simulink model "player_ball_5"  (R2021b)
settings: Solver=VariableStepAuto  StartTime=0.0  StopTime=300  RelTol=1e-3
model workspace (MAT data in the model file):
  trailfuzzy = 'trailfuzzy.fis'
values from neighbouring files (symbols this model uses):
  initBallPos = fieldCenter    [robotSoccerParams.m]
  robotDetectorMaxHits = 5    [robotSoccerParams.m]
  sampleTime = 0.05    [robotSoccerParams.m]
undefined symbols (not defined in the file or in its folder): DiscIntNeverNeededParam
libraries: mobileRoboticsLib x11, dspindex x3, fuzblock x2
settings Model: Creator=kstkr  LastModifiedBy=kstkr
settings DebuggingCC: AlgebraicLoopMsg=none

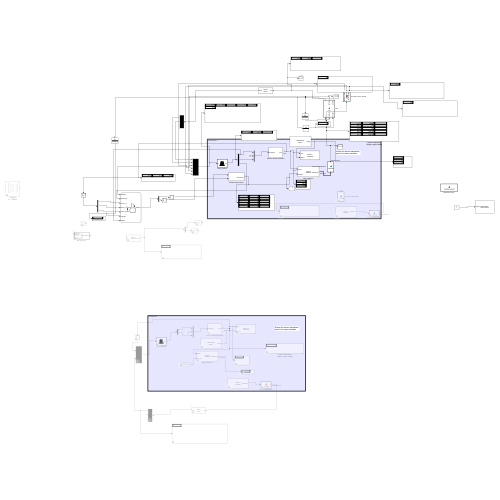
[thumbnail: Simulink's stored preview of the top-level diagram]
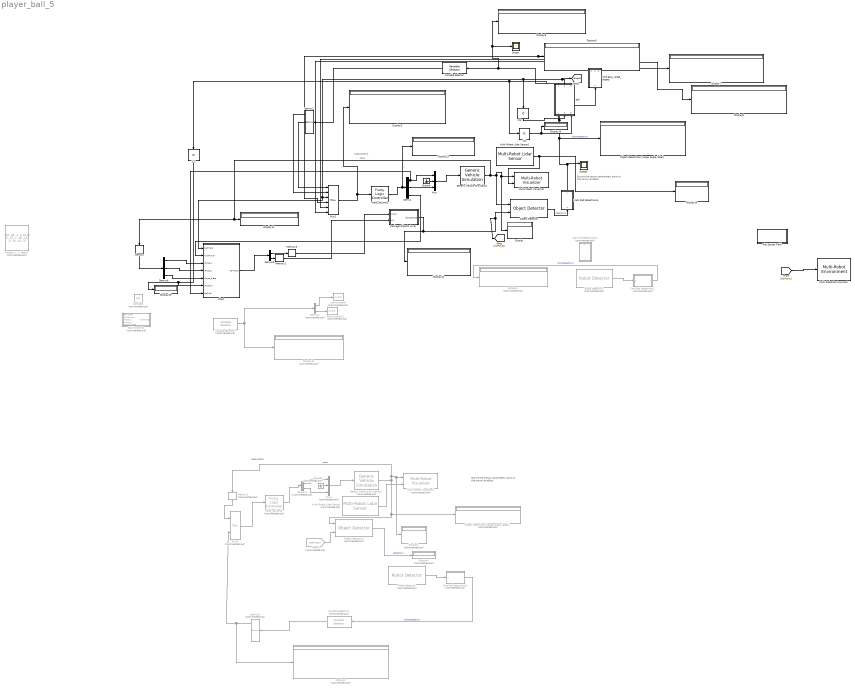
== system player_ball_5 ==
  note: Subsystem1
  note: Subsystem
  note: Ensure the sensor parameters point to the same variables.
  note: Ensure the sensor parameters point to the same variables.
  Add Constant : Bias  Commented=on  Bias=0.3
  Add Constant1 : Bias  Commented=on  Bias=0.3
  Ball Dynamics : MATLAB Function  Commented=on  TreatAsAtomicUnit=on
  Chart : Stateflow chart  TreatAsAtomicUnit=on
  Constant : Constant  Commented=on  Value=0.5
  Demux : Demux  Outputs=3
  Demux1 : Demux  Commented=on  Outputs=2
  Demux2 : Demux  Outputs=3
  Demux3 : Demux  Commented=on  Outputs=3
  Demux4 : Demux  Commented=on  Outputs=2
  Demux5 : Demux  Outputs=2
  Demux6 : Demux  Outputs=3
  Display{,3,6..9,11..16} (12 alike) : Display
  Display{1..2,4..5,10} (5 alike) : Display  Commented=on
  From1 : From  Commented=on  GotoTag=objPoses
  Generic Vehicle Simulation : mobileRoboticsLib/Utilities/Generic Vehicle Simulation  initX=6  initY=8  initAngle=0  Ts=sampleTime
      settings: SourceProductName=Mobile Robotics Simulation Library
  Generic Vehicle Simulation1 : mobileRoboticsLib/Utilities/Generic Vehicle Simulation  Commented=on  initX=80  initY=10  initAngle=pi  Ts=sampleTime
      settings: SourceProductName=Mobile Robotics Simulation Library
  Ground : Ground
  Ground1 : Ground  Commented=on
  IC1 : InitialCondition
  IC2 : InitialCondition  Value=0
  IC3 : InitialCondition  Value=0
  Memory : Memory  InitialCondition=[15 2 0]  InheritSampleTime=on
  Memory1 : Memory  Commented=on  InitialCondition=[15 2 0]
  Memory2 : Memory  InheritSampleTime=on  LinearizeAsDelay=on
  Memory3 : Memory  InheritSampleTime=on  LinearizeAsDelay=on
  Multi-Robot Environment : mobileRoboticsLib/Environments/Multi-Robot Environment  numRobots=1  mapName=map  showWaypoints=off  showObjects=on  objectColors=objColors  objectMarkers=objMarkers  showRobotIds=on  plotSensorLines=on
      settings: SourceProductName=Mobile Robotics Simulation Toolbox
  Multi-Robot Lidar Sensor : mobileRoboticsLib/Environments/Multi-Robot Lidar Sensor  Commented=on  robotIdx=1  mapName=map  sensorOffset=[0,0]  scanAngles=[-pi/4 0 pi/4]  maxRange=20
      settings: SourceProductName=Mobile Robotics Simulation Toolbox
  Multi-Robot Lidar Sensor1 : mobileRoboticsLib/Environments/Multi-Robot Lidar Sensor  robotIdx=1  mapName=map  sensorOffset=[0,0]  scanAngles=[-pi/4 0 pi/4]  maxRange=5
      settings: SourceProductName=Mobile Robotics Simulation Toolbox
  Multi-Robot Visualizer : mobileRoboticsLib/Environments/Multi-Robot Visualizer  idx=1  radius=1  robotColor=[0 0 1]  showTraj=on  hasLidar=on  sensorOffset=[0,0]  scanAngles=[-pi/4 0 pi/4]  maxNumScans=0  hasObjDetector=off  objDetectorOffset=[0,0]  objDetectorAngle=0  objDetectorFOV=pi/3  objDetectorMaxRange=5  hasRobotDetector=off  robotDetectorOffset=[0,0]  robotDetectorAngle=0  robotDetectorFOV=pi/3  robotDetectorMaxRange=5  robotDetectorNumDetections=0
      settings: SourceProductName=Mobile Robotics Simulation Toolbox
  Multi-Robot Visualizer1 : mobileRoboticsLib/Environments/Multi-Robot Visualizer  Commented=on  idx=2  radius=1  robotColor=[1 0 0]  showTraj=on  hasLidar=on  sensorOffset=[0,0]  scanAngles=[-pi/4 0 pi/4]  maxNumScans=0  hasObjDetector=off  objDetectorOffset=[0,0]  objDetectorAngle=0  objDetectorFOV=pi/3  objDetectorMaxRange=5  hasRobotDetector=off  robotDetectorOffset=[0,0]  robotDetectorAngle=0  robotDetectorFOV=pi/3  robotDetectorMaxRange=5  robotDetectorNumDetections=0
      settings: SourceProductName=Mobile Robotics Simulation Toolbox
  Mux : Mux  Inputs=3
  Mux1 : Mux  Commented=on  Inputs=3
  Mux2 : Mux  Inputs=6
  Mux3 : Mux  Commented=on  Inputs=2
  "Object Detections [range, angle, label]" : Display
  "Object Detections [range, angle, label]1" : Display  Commented=on
  Object Detector : mobileRoboticsLib/Environments/Object Detector  mapName=map  sensorOffset=objDetectorOffset  sensorAngle=objDetectorAngle  fieldOfView=objDetectorFOV  maxRange=objDetectorRange  maxDetections=objDetectorMaxHits  sampleTime=-1
      settings: SourceProductName=Ground Vehicles Library
  Object Detector1 : mobileRoboticsLib/Environments/Object Detector  Commented=on  mapName=map  sensorOffset=objDetectorOffset  sensorAngle=objDetectorAngle  fieldOfView=objDetectorFOV  maxRange=objDetectorRange  maxDetections=objDetectorMaxHits  sampleTime=-1
      settings: SourceProductName=Ground Vehicles Library
  "Objects [x, y, label]1" : Constant  Commented=on  Value=[45, 30, 1; 0,15,2; 0, 45, 2; 90, 15, 3; 90, 45, 3]
  Package Objects Array : Subsystem
  Plot Soccer Field : MATLAB Function  TreatAsAtomicUnit=on
  Robot Detector : mobileRoboticsLib/Environments/Robot Detector  Commented=on  mapName=map  robotIdx=2  sensorOffset=robotDetectorOffset  sensorAngle=robotDetectorAngle  sensorFOV=pi/3  maxRange=100  maxDetections=robotDetectorMaxHits  sampleTime=sampleTime
      settings: SourceProductName=Mobile Robotics Simulation Toolbox
  Robot Detector1 : mobileRoboticsLib/Environments/Robot Detector  Commented=on  mapName=map  robotIdx=1  sensorOffset=robotDetectorOffset  sensorAngle=robotDetectorAngle  sensorFOV=pi/3  maxRange=100  maxDetections=robotDetectorMaxHits  sampleTime=sampleTime
      link override Robot Detector: mapName=map  maxDetections=5
      settings: SourceProductName=Mobile Robotics Simulation Toolbox
  Scope : Scope
  Scope2 : Scope  NumInputPorts=2
  Variable Selector : dspindex/Variable Selector  NumInputs=1  rowsOrCols=Rows  IdxMode=Fixed  Elements="[1  ]"  ZerOneIdxMode=One-based  errmode=Clip Index  FillMode=off  FillValues=0
  Variable Selector1 : dspindex/Variable Selector  Commented=on  NumInputs=1  rowsOrCols=Rows  IdxMode=Fixed  Elements="[1  ]"  ZerOneIdxMode=One-based  errmode=Clip Index  FillMode=off  FillValues=0
  Variable Selector2 : dspindex/Variable Selector  Commented=on  NumInputs=1  rowsOrCols=Columns  IdxMode=Fixed  Elements=[1 2]  ZerOneIdxMode=One-based  errmode=Clip Index  FillMode=on  FillValues=0
  Zero Pad Detections1 : MATLAB Function  Commented=on  TreatAsAtomicUnit=on  mask(Zero Pad Detections){maxHits=robotDetectorMaxHits}
      mask prompts: maxHits "Maximum Sensor Hits"
      mask help: Zero pads detections matrix so it is fixed-size and works with arrays of buses.
  Zero Pad Detections2 : MATLAB Function  Commented=on  TreatAsAtomicUnit=on  mask(Zero Pad Detections){maxHits=robotDetectorMaxHits}
      mask prompts: maxHits "Maximum Sensor Hits"
      mask help: Zero pads detections matrix so it is fixed-size and works with arrays of buses.
  Zero Pad Detections3 : MATLAB Function  Commented=on  TreatAsAtomicUnit=on  mask(Zero Pad Detections){maxHits=robotDetectorMaxHits}
      mask prompts: maxHits "Maximum Sensor Hits"
      mask help: Zero pads detections matrix so it is fixed-size and works with arrays of buses.
  Zero Pad Detections4 : MATLAB Function  TreatAsAtomicUnit=on  mask(Zero Pad Detections){maxHits=robotDetectorMaxHits}
      mask prompts: maxHits "Maximum Sensor Hits"
      mask help: Zero pads detections matrix so it is fixed-size and works with arrays of buses.
  ball : MATLAB Function  TreatAsAtomicUnit=on
  idx3 goal_range_angles : MATLAB Function  TreatAsAtomicUnit=on
  robot_actions1 : fuzblock/Fuzzy Logic  Controller  FIS='A1trialfuzzyball3.fis'  OutputSampleNumber=101  DataType=double  FuzzifiedInputs=off  RuleFiringStrengths=off  RuleOutputs=off  AggregatedOutputs=off  SimulateUsing=Interpreted execution  OutOfRangeInputValueMessage=warning  NoRuleFiredMessage=warning  EmptyOutputFuzzySetMessage=warning
  robot_actions2 : fuzblock/Fuzzy Logic  Controller  Commented=on  FIS='trialfuzzy2_2.fis'  OutputSampleNumber=101  DataType=double  FuzzifiedInputs=off  RuleFiringStrengths=off  RuleOutputs=off  AggregatedOutputs=off  SimulateUsing=Interpreted execution  OutOfRangeInputValueMessage=warning  NoRuleFiredMessage=warning  EmptyOutputFuzzySetMessage=warning
  wires:
  Robot Detector/1 -> Zero Pad Detections1/1(u)
  Demux1/1 -> Mux1/1
  Ground1/1 -> Mux1/2
  robot_actions2/1 -> Demux1/1  "v"
  Mux1/1 -> Generic Vehicle Simulation1/1
  Mux3/1 -> robot_actions2/1
  Demux1/2 -> Mux1/3
  Generic Vehicle Simulation1/1 -> Memory1/1, Display1/1, Multi-Robot Visualizer1/1, Object Detector1/1, "Object Detections [range, angle, label]1"/1  "pose"
  Robot Detector1/1 -> Zero Pad Detections2/1(u)
  Zero Pad Detections2/1(y) -> Display5/1  "robotDetections"
  Mux/1 -> Generic Vehicle Simulation/1
  Ground/1 -> Mux/2
  robot_actions1/1 -> Display13/1, Demux/1  "v"
  Demux/1 -> Chart/7(ballVel), Mux/1
  Demux/2 -> Mux/3
  Generic Vehicle Simulation/1 -> Memory/1, Display11/1, Object Detector/1, Display/1, Multi-Robot Visualizer/1  "pose"
  Mux2/1 -> Display3/1, robot_actions1/1
  Object Detector/1 -> Zero Pad Detections4/1(u)  "detections"
  Memory1/1 -> Mux3/1
  Variable Selector/1 -> Demux2/1
  Demux2/1 -> Mux2/2
  Zero Pad Detections1/1(y) -> Variable Selector1/1  "robotDetections"
  Variable Selector1/1 -> Demux3/1
  Demux3/1 -> Display2/1, Mux3/2
  Multi-Robot Lidar Sensor/1 -> Multi-Robot Visualizer1/2
  Multi-Robot Lidar Sensor1/1 -> Display16/1, Multi-Robot Visualizer/2
  [objPoses] -> Multi-Robot Environment/1
  Object Detector1/1 -> Display4/1  "detections"
  From1/1 -> Object Detector1/2
  Demux2/2 -> Mux2/1
  Zero Pad Detections4/1(y) -> Scope2/1, "Object Detections [range, angle, label]"/1, idx3 goal_range_angles/1(u), ball/1(u)  "robotDetections"
  ball/1(y) -> Scope/1, Display9/1, Variable Selector/1
  idx3 goal_range_angles/1(goalRight_angle) -> Mux2/4, Display6/1
  idx3 goal_range_angles/2(goalRange) -> Mux2/5, Display7/1
  idx3 goal_range_angles/3(goalLeft_angle) -> Mux2/6, Display8/1
  Variable Selector2/1 -> Demux4/1, Display10/1
  Demux4/1 -> Add Constant/1
  Demux4/2 -> Add Constant1/1
  Demux5/1 -> Memory3/1
  Demux5/2 -> Memory2/1
  Memory/1 -> Demux6/1
  Memory3/1 -> Package Objects Array/1(Inport)
  Memory2/1 -> Package Objects Array/2(In2)
  Demux6/1 -> Chart/3(rPose_x)
  Demux6/2 -> Chart/4(rPose_y)
  Demux6/3 -> Chart/5(rPose_theta)
  Demux/3 -> Chart/2(KickPower)
  Chart/1(ballPose) -> Demux5/1
  ball/3(robotIdx) -> IC2/1, IC1/1
  IC1/1 -> Chart/6(robotIdx), Display15/1
  ball/2(ballHeld) -> IC3/1, Chart/1(ballHeld), Mux2/3, [bheld]
  IC2/1 -> Display14/1, ball/3("robotIdx ")
  IC3/1 -> ball/2("ballHeld ")
  Package Objects Array/1(objectsPose) -> Object Detector/2, [objPoses], Display12/1

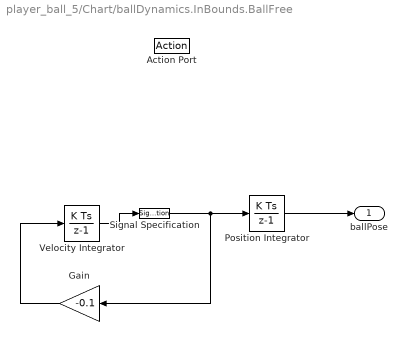
== system player_ball_5/Chart/ballDynamics.InBounds.BallFree ==
  Action Port : ActionPort
      settings: CopyFcn=Stateflow.SLINSF.SimulinkMan.removeBlockPreDeleteFcn  PreDeleteFcn=Stateflow.SLINSF.SimulinkMan.unsafePredeleteFcn
  Gain : Gain  Gain=-0.1
  Position Integrator : DiscreteIntegrator  InitialCondition=initBallPos  SampleTime=-1  StateName=ballPos  ICPrevOutput=DiscIntNeverNeededParam  ICPrevScaledInput=DiscIntNeverNeededParam
  Signal Specification : SignalSpecification  Dimensions=[1 2]
  Velocity Integrator : DiscreteIntegrator  InitialCondition=[0 0]  SampleTime=-1  StateName=ballVel  ICPrevOutput=DiscIntNeverNeededParam  ICPrevScaledInput=DiscIntNeverNeededParam
  ballPose : Outport  VectorParamsAs1DForOutWhenUnconnected=off
  wires:
  Signal Specification/1 -> Gain/1, Position Integrator/1
  Position Integrator/1 -> ballPose/1
  Velocity Integrator/1 -> Signal Specification/1
  Gain/1 -> Velocity Integrator/1

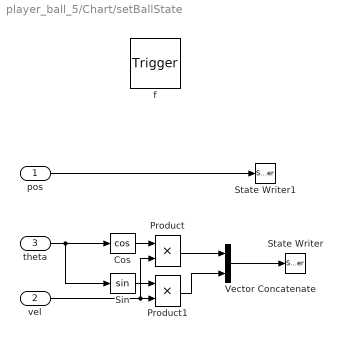
== system player_ball_5/Chart/setBallState ==
  pos : Inport  OutDataTypeStr=double  PortDimensions=[1 2]
  vel : Inport  Port=2  OutDataTypeStr=double  PortDimensions=1
  theta : Inport  Port=3  OutDataTypeStr=double  PortDimensions=1
  f : TriggerPort  TriggerType=function-call  VariantControl=(inherit)
      settings: CopyFcn=Stateflow.SLINSF.SimulinkMan.removeBlockPreDeleteFcn  PreDeleteFcn=Stateflow.SLINSF.SimulinkMan.unsafePredeleteFcn
  Cos : Trigonometry  Operator=cos
  Product : Product
  Product1 : Product
  Sin : Trigonometry
  State Writer : StateWriter  StateOwnerBlock=../../ballDynamics.InBounds.BallFree/Velocity Integrator  StateName=ballVel
  State Writer1 : StateWriter  StateOwnerBlock=../../ballDynamics.InBounds.BallFree/Position Integrator  StateName=ballPos
  Vector Concatenate : Concatenate  Mode=Multidimensional array  ConcatenateDimension=2
  wires:
  Sin/1 -> Product1/1
  Product1/1 -> Vector Concatenate/2
  Product/1 -> Vector Concatenate/1
  theta/1 -> Cos/1, Sin/1
  vel/1 -> Product1/2, Product/2
  Cos/1 -> Product/1
  Vector Concatenate/1 -> State Writer/1
  pos/1 -> State Writer1/1

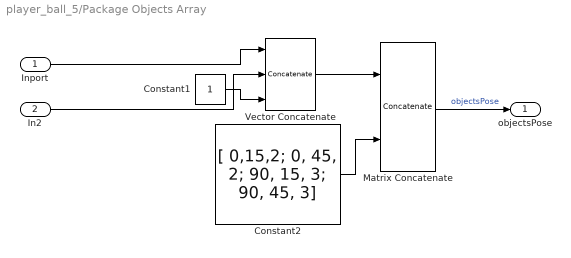
== system player_ball_5/Package Objects Array ==
  Inport : Inport
  In2 : Inport  Port=2
  Constant1 : Constant
  Constant2 : Constant  Value=[ 0,15,2; 0, 45, 2; 90, 15, 3; 90, 45, 3]
  Matrix Concatenate : Concatenate  Mode=Multidimensional array
  Vector Concatenate : Concatenate  NumInputs=3  Mode=Multidimensional array  ConcatenateDimension=2
  objectsPose : Outport  VectorParamsAs1DForOutWhenUnconnected=off
  wires:
  Vector Concatenate/1 -> Matrix Concatenate/1
  Matrix Concatenate/1 -> objectsPose/1  "objectsPose"
  Constant2/1 -> Matrix Concatenate/2
  Inport/1 -> Vector Concatenate/1
  Constant1/1 -> Vector Concatenate/3
  In2/1 -> Vector Concatenate/2

== matlab function player_ball_5/Zero Pad Detections3 ==
  data: u input size=[maxHits 3]; y output size=[maxHits 3]; maxHits parameter
function y = zeroPad(u,maxHits)
% Zero-pads object detections to work with arrays of buses

y = zeros(maxHits,3);
numElems = min(size(u,1),maxHits);
for idx = 1:numElems
   y(idx,1:3) = u(idx,1:3); 
end

== matlab function player_ball_5/ball ==
  data: u input; y output; ballHeld output; robotIdx output; ballHeld input; robotIdx input

function [y,ballHeld, robotIdx]= fcn(u,ballHeld,robotIdx)
a = u(1,:);
b = u(2,:);
c = u(3,:);
d = u(4,:);
e = u(5,:);
if a(3) ==1
    y = a;


elseif b(3) ==1
    y = b;


elseif c(3)==1
    y=c;


elseif d(3)==1
    y=d;


else
    y = e;


end
if y(1)  <= 1.1
    ballHeld = 1;
    robotIdx =1;

else
    ballHeld =0;
    robotIdx =0;

end

== matlab function player_ball_5/Ball Dynamics ==
  data: ballPose output; ballHeld input; KickPower input; rPose_x input; rPose_y input; rPose_theta input
function ballPose  = fcn(ballHeld, KickPower,rPose_x, rPose_y, rPose_theta)
ballPose = [25 10];
if ballHeld == 1 
    ballPose = [rPose_x rPose_y] + (0.8 + 0.3)*[cos(rPose_theta) sin(rPose_theta)];

elseif KickPower >= 5.5 && ballHeld == 1
    %ballPose = KickPower*[rPose_x rPose_y] + (0.8 + 0.3)*[cos(rPose_theta) sin(rPose_theta)];
    ballHeld = 0
    ballPose = KickPower*[rPose_x rPose_y] + (0.8 + 0.3)*[cos(rPose_theta) sin(rPose_theta)];
    %if KickPower ~=0
    %    ballPose = KickPower*[rPose_x rPose_y] + (0.8 + 0.3)*[cos(rPose_theta) sin(rPose_theta)];
    %end

end

== matlab function player_ball_5/Zero Pad Detections1 ==
  data: u input size=[maxHits 3]; y output size=[maxHits 3]; maxHits parameter
function y = zeroPad(u,maxHits)
% Zero-pads object detections to work with arrays of buses

y = zeros(maxHits,3);
numElems = min(size(u,1),maxHits);
for idx = 1:numElems
   y(idx,1:3) = u(idx,1:3); 
end

== matlab function player_ball_5/idx3 goal_range_angles ==
  data: u input; goalRight_angle output; goalRange output; goalLeft_angle output
% function y = fcn(u)
% for i = 1:5
%     if u(i,3) == 1
%         a = u(i,:)
%     end
% end
% % b = u(2,:)
% % c = u(3,:)
% % d = u(4,:)
% % e = u(5,:)
% y = a;
% end
%two indexes are same. How to identify right and left angles
% for now randomly assigned the values
% goal range is minimum of the two 


function [goalRight_angle,goalRange, goalLeft_angle]= fcn(u)
goalRight_angle=0;
goalLeft_angle=0;
right_range = 0;
left_range =0;
k=0;
for i= 1:5
    if u(i,3) == 3 && k==0
        goalRight_angle = u(i,2);
        right_range = u(i,1);
        k = k+1;
    elseif u(i,3) ==3 && k==1
        goalLeft_angle = u(i,2);
        left_range = u(i,1);
        k =0;

    end

end
if right_range < left_range
    goalRange = right_range;
else
    goalRange = left_range;
end


end

== matlab function player_ball_5/Zero Pad Detections4 ==
  data: u input size=[maxHits 3]; y output size=[maxHits 3]; maxHits parameter
function y = zeroPad(u,maxHits)
% Zero-pads object detections to work with arrays of buses

y = zeros(maxHits,3);
numElems = min(size(u,1),maxHits);
for idx = 1:numElems
   y(idx,1:3) = u(idx,1:3); 
end

== stateflow chart player_ball_5/Chart ==
  state ballDynamics
    en:
    coder.extrinsic('randn');
    setBallState([45 30],0,0);
    state InBounds
      en:
      randNum = randn(2,1);
      state BallFree
      state BallHeld
        en,du:
        ballPose = [rPose_x rPose_y] + ...
        (0.8+0.3)*[cos(rPose_theta) sin(rPose_theta)];
      (default) -> BallFree
      BallHeld -> BallFree : [KickPower>7]{setBallState(ballPose,KickPower*10*ballVel, ...
          |  rPose_theta)}
      BallFree -> BallHeld : [after(2,sec) && ...
          |  ballHeld > 0]
    state Outofbounds
      en:
      ballPose = [45 30];
      setBallState(ballPose,0,rPose_theta)
    (default) -> InBounds
    Outofbounds -> InBounds : [after(1,sec)]
    InBounds -> Outofbounds : [ballPose(1) > 90]
  state setBallState(pos,vel,theta) [function]
  data: sf_internal_action_state_placeholder_data local double size=1 =0; pos function_input double size=[1 2]; vel function_input double size=1; theta function_input double size=1; ballHeld input; KickPower input; rPose_x input; rPose_y input; rPose_theta input; robotIdx input; ballPose output; randNum local; action local; ballVel input

== matlab function player_ball_5/Zero Pad Detections2 ==
  data: u input size=[maxHits 3]; y output size=[maxHits 3]; maxHits parameter
function y = zeroPad(u,maxHits)
% Zero-pads object detections to work with arrays of buses

y = zeros(maxHits,3);
numElems = min(size(u,1),maxHits);
for idx = 1:numElems
   y(idx,1:3) = u(idx,1:3); 
end

== matlab function player_ball_5/Plot Soccer Field ==
function plotSoccerField
% Plots the soccer field once the figure window for the environment has
% been initialized

coder.extrinsic('evalin');
persistent hasPlotted
if isempty(hasPlotted)
    evalin('base','plotSoccerField');
    hasPlotted = true;
end
